simulink model "Foc_model_Matlab"  (R2024b)
settings: Solver=FixedStepDiscrete  StartTime=0.0  StopTime=2  RelTol=1e-3  EnableMultiTasking=on
PreLoadFcn:
  | mcb_pmsm_foc_hall_S32K144EVB_data;
InitFcn:
  | mbd_s32k_consistency_checks(bdroot(gcs));
model workspace (MAT data in the model file):
  IDC_OVERCURRENT = Simulink.Parameter
  IDC_OVERCURRENT.Value = 2.3
  IDC_OVERCURRENT.Complexity = 'real'
  IDC_OVERCURRENT.Dimensions = [1 1]
  IDC_OVERCURRENT.DataType = 'single'
  VDC_OVERVOLTAGE = Simulink.Parameter
  VDC_OVERVOLTAGE.Value = 16
  VDC_OVERVOLTAGE.Complexity = 'real'
  VDC_OVERVOLTAGE.Dimensions = [1 1]
  VDC_OVERVOLTAGE.DataType = 'single'
  VDC_UNDERVOLTAGE = Simulink.Parameter
  VDC_UNDERVOLTAGE.Value = 8
  VDC_UNDERVOLTAGE.Complexity = 'real'
  VDC_UNDERVOLTAGE.Dimensions = [1 1]
  VDC_UNDERVOLTAGE.DataType = 'single'
values from neighbouring files (symbols this model uses):
  Kcd = (1/pmsm.p)*(2*zeta1*wnd*pmsm.Ld)-pmsm.Rs    [Foc_data.m]
  Kcq = (2*zeta1*wnq*pmsm.Lq)-pmsm.Rs    [Foc_data.m]
  Kcs = (1/pmsm.p)*(2*zeta2*wns-(pmsm.B/pmsm.J))/((1.5*pmsm.p^2*pmsm.FluxPM)/pmsm.J)    [Foc_data.m]
  Kid = Kcd/t_id    [Foc_data.m]
  Kiq = Kcq/t_iq    [Foc_data.m]
  Kis = Kcs/t_is    [Foc_data.m]
  Ts = T_pwm * 2    (= 0.0001)    [Foc_data.m]
  Ts_motor = T_pwm    (= 5e-05)    [Foc_data.m]
  Ts_simulink = T_pwm    (= 5e-05)    [Foc_data.m]
  Ts_speed = 10*Ts    (= 0.001)    [Foc_data.m]
undefined symbols (not defined in the file or in its folder): External, inverter, LQFP, mcb_isCodeGenVar, mcb_isSimVar, One, PI_params, pmsm, PU_System, Shot, TRGMUX_PDB_TRIG
libraries: mbd_s32k1xx_ec_toolbox x39, mcbcontrolslib x9, simulink x6, mcbpositiondecoderlib x5, mbd_msd_ec_toolbox x5, hdlsllib x4, mcbplantlib x1, autolibpmsmexterior x1, SignalEditorBlockLib x1
(part 1 of 2)
Description:
  | Field-Oriented Control for PMSM with Hall sensor with MTRDEVSPNK144.
  | This Simulink model is designed to work with Linix 45ZWN24-40 Motor and validate
  | that the motor can be rotated in closed loop with Hall sensor in Mathworks model from Motor Control Blockset.
  | The main scope of the model is to validate that the motor can run using Field-Oriented Control with Hall sensor.
  | 
  | FEATURES:
  | - Use FreeMASTER pannel to control the speed,
  | - Measure the 3-phase sinusoidal currents with PWM-PDB-ADC synchronization,
  | - Measure the DC bus voltage and current with PWM-PDB-ADC synchronization,
  | - PI Speed, Flux and Torque Controllers, position observer using Hall sensor.
  | 
  | HW SETUP:
  | - Configure S32K144 board supply voltage: J107:2-3(over USB),
  | - Configure J9,J10 and J11 on MotorGD: 2-3 (mode PMSM),
  | - Rotate trimmer resistor R72 (placed Devkit-MotorGD) counter-clockwise at maximum,
  | - Connect the motor phases to MotorGD J13 connector
  |   (i.e. Linix 45ZWN24-40: phA-white/phB-blue/phC-green),
  | - Power on the kit via J7 connector with 12Vdc.
  | 
  | VALIDATION:
  | - Run "mcb_pmsm_hall_offset_S32K144EVB_NXP.mdl" model to find out the position offset and
  | update it in "mcb_pmsm_foc_hall_S32K144EVB_data.m" script, run this script,
  | - Build/Simulate the model,
  | - After reset or power on, the Green LED shall be ON,
  | - In case of a FAULT the Red LED will be ON,
  | - Open FreeMASTER project and connect to the target.
  | - The initial speed command is set to 450rpm and can be changed from FreeMaster project.
  | - Click on the ON/OFF button to start then the speed of the motor it can be
  | changed using Speed gauge.
  | 
  | NOTE:
  | - In case of fault (RED LED is ON), the remove fault cause and press RESET button
  | 
  | Copyright (c) 2021 NXP
  | version 1.0.0
settings Model: Creator=nxf40284  LastModifiedBy=diego
settings SolverCC: AlgebraicLoopSolver=TrustRegion
settings DataIOCC: ExternalInput=off  InitialState=off  LimitDataPoints=on  SaveFormat=Array  SaveOutput=off  SaveTime=off  ReturnWorkspaceOutputs=off
settings OptimizationCC: DefaultParameterBehavior=Inlined  UseFloatMulNetSlope=on  DefaultUnderspecifiedDataType=single  UseSpecifiedMinMax=on  EnhancedBackFolding=on  PassReuseOutputArgsAs=Individual arguments  ZeroExternalMemoryAtStartup=off  ZeroInternalMemoryAtStartup=off  NoFixptDivByZeroProtection=on  EfficientFloat2IntCast=on  EfficientTunableParamExpr=on
settings DebuggingCC: AlgebraicLoopMsg=error  ArtificialAlgebraicLoopMsg=error  SolverPrmCheckMsg=warning  InheritedTsInSrcMsg=none  MultiTaskDSMMsg=none  MultiTaskCondExecSysMsg=none  TasksWithSamePriorityMsg=none  SigSpecEnsureSampleTimeMsg=none  ParameterPrecisionLossMsg=none  ParameterTunabilityLossMsg=error  FcnCallInpInsideContextMsg=warning  UnconnectedInputMsg=error  UnconnectedOutputMsg=error  UnconnectedLineMsg=error  AllowSymbolicDim=off  StateNameClashWarn=warning  SFUnexpectedBacktrackingDiag=warning  SFNoUnconditionalDefaultTransitionDiag=warning  SFExecutionAtInitializationDiag=none  ArithmeticOperatorsInVariantConditions=warning
settings HardwareCC: ProdBitPerPointer=32  ProdBitPerSizeT=32  ProdBitPerPtrDiffT=32  ProdLargestAtomicInteger=Long  ProdLargestAtomicFloat=Double  ProdWordSize=32  ProdHWDeviceType=ARM Compatible->ARM Cortex
settings ModelReferenceCC: EnableRefExpFcnMdlSchedulingChecks=on
settings SFSimCC: MATLABDynamicMemAlloc=off
settings RTWCC: Description=Model Based Design Toolbox S32K1xx Code Generation Target  SystemTargetFile=mbd_s32k.tlc  MakeCommand=mbd_s32k_make_rtw COPY_MDLREF_INCLUDES=0  TemplateMakefile=mbd_s32k.tmf  GenerateReport=on  IncludeHyperlinkInReport=on  GenerateTraceInfo=on  GenerateTraceReport=on  GenerateTraceReportSl=on  GenerateTraceReportSf=on  GenerateTraceReportEml=on  GPUComputeCapability=3.5
settings CodeAppCC: ForceParamTrailComments=on  IgnoreCustomStorageClasses=off  OperatorAnnotations=on  SimulinkDataObjDesc=on  SFDataObjDesc=on  InsertBlockDesc=on  StateflowObjectComments=on
settings STFCustomTargetCC: MultiwordLength=256  CombineOutputUpdateFcns=on  ERTCustomFileBanners=on  SupportContinuousTime=off  SupportNonInlinedSFcns=off  RemoveResetFunc=on  MATLABClassNameForMDSCustomization=Simulink.SoftwareTarget.ERTCustomization  SystemTargetFile=mbd_s32k.tlc
settings ERTTargetCC: ParMdlRefBuildCompliant=off  CompOptLevelCompliant=off  ConcurrentExecutionCompliant=off  ModelStepFunctionPrototypeControlCompliant=off  CPPClassGenCompliant=off  UseToolchainInfoCompliant=off  ERTSrcFileBannerTemplate=mbd_ert_code_template.cgt  ERTHdrFileBannerTemplate=mbd_ert_code_template.cgt  ERTDataSrcFileTemplate=mbd_ert_code_template.cgt  ERTDataHdrFileTemplate=mbd_ert_code_template.cgt  ERTCustomFileTemplate=example_file_process.tlc  ConvertIfToSwitch=off  SuppressUnreachableDefaultCases=off  DynamicArrayContainerType=coder::array

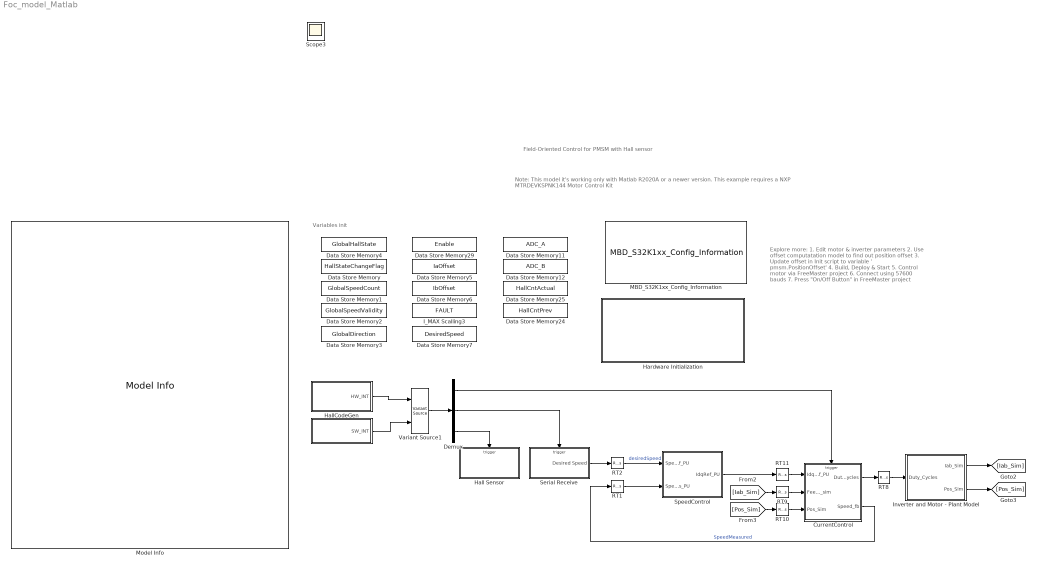
== system Foc_model_Matlab ==
  note: Variables init
  note: Field-Oriented Control for PMSM with Hall sensor
  note: Explore more:
      | 1. Edit motor & inverter parameters
      | 2. Use offset computatation model to
      | find out position offset
      | 3. Update offset in Init script to variable ' pmsm.PositionOffset'
      | 4. Build, Deploy & Start
      | 5. Control motor via FreeMaster project
      | 6. Connect using 57600 bauds
      | 7. Press "On/Off Button" in FreeMaster project
  note: Note: This model it's working only with Matlab R2020A or a newer version.
      | This example requires a NXP MTRDEVKSPNK144 Motor Control Kit
  " " : Subsystem
  CurrentControl : Subsystem
      settings: RTWSystemCode=Nonreusable function  RTWFcnNameOpts=Use subsystem name
  Data Store Memory : DataStoreMemory  DataStoreName=HallStateChangeFlag  ShowAdditionalParam=off  OutDataTypeStr=uint16
  Data Store Memory1 : DataStoreMemory  DataStoreName=GlobalSpeedCount  ShowAdditionalParam=off  OutDataTypeStr=uint16
  Data Store Memory11 : DataStoreMemory  DataStoreName=ADC_A  ShowAdditionalParam=off
  Data Store Memory12 : DataStoreMemory  DataStoreName=ADC_B  ShowAdditionalParam=off
  Data Store Memory2 : DataStoreMemory  DataStoreName=GlobalSpeedValidity  ShowAdditionalParam=off  OutDataTypeStr=uint16
  Data Store Memory24 : DataStoreMemory  DataStoreName=HallCntPrev  ReadBeforeWriteMsg=warning  WriteAfterWriteMsg=warning  WriteAfterReadMsg=warning  ShowAdditionalParam=off  OutDataTypeStr=uint16
  Data Store Memory25 : DataStoreMemory  DataStoreName=HallCntActual  ReadBeforeWriteMsg=warning  WriteAfterWriteMsg=warning  WriteAfterReadMsg=warning  ShowAdditionalParam=off  OutDataTypeStr=uint16
  Data Store Memory29 : DataStoreMemory  DataStoreName=Enable  ShowAdditionalParam=off  OutDataTypeStr=boolean
  Data Store Memory3 : DataStoreMemory  DataStoreName=GlobalDirection  ShowAdditionalParam=off  OutDataTypeStr=int16
  Data Store Memory4 : DataStoreMemory  DataStoreName=GlobalHallState  ShowAdditionalParam=off  OutDataTypeStr=uint32
  Data Store Memory5 : DataStoreMemory  DataStoreName=IaOffset  InitialValue=inverter.CtSensAOffset  ShowAdditionalParam=off  OutDataTypeStr=single
  Data Store Memory6 : DataStoreMemory  DataStoreName=IbOffset  InitialValue=inverter.CtSensBOffset  ShowAdditionalParam=off  OutDataTypeStr=single
  Data Store Memory7 : DataStoreMemory  DataStoreName=DesiredSpeed  ReadBeforeWriteMsg=warning  WriteAfterWriteMsg=warning  WriteAfterReadMsg=warning  InitialValue=450  ShowAdditionalParam=off  OutDataTypeStr=single
  Demux : Demux  Outputs=3
  Hall Sensor : Subsystem
  HallCodeGen : Subsystem
  Hardware Initialization : Subsystem  Priority=2
  I_MAX Scalling3 : DataStoreMemory  Priority=0  DataStoreName=FAULT  ReadBeforeWriteMsg=warning  WriteAfterWriteMsg=warning  WriteAfterReadMsg=warning  ShowAdditionalParam=off  OutDataTypeStr=boolean
  Inverter and Motor - Plant Model : Subsystem
  MBD_S32K1xx_Config_Information : mbd_s32k1xx_ec_toolbox/MBD_S32K1xx_Config_Information  Priority=1  mbdt_ver=0  disp_str=|  config_params=[]  mcu_target_name=S32K144  mcu_target_package=100-LQFP  mcu_target_sram_size=64KB  mcu_system_clock_freq=80  mcu_xtal_freq=External 8  mcu_steptick_timer=LPIT Channel 0  mcu_steptick_prio=15  ds_import_enable=on  target_compiler=GCC  target_memory=FLASH  gcc_target_compile_opts=-mcpu=cortex-m4 -mthumb -mfloat-abi=hard -mfpu=fpv4-sp-d16 -O1 -g -gstrict-dwarf  gcc_target_assemble_opts=-mcpu=cortex-m4 -mthumb -mfloat-abi=hard -mfpu=fpv4-sp-d16 -g  gcc_target_link_opts=-mcpu=cortex-m4 -mthumb -mfloat-abi=hard -mfpu=fpv4-sp-d16  gcc_target_default_lcf=on  gcc_target_user_lcf=S32K144_64_flash.ld  ghs_target_compile_opts=-cpu=cortexm4f -thumb -DARM_MATH_CM4 -fpu=vfpv4_d16 -fsingle -Ogeneral -Wundef -Wimplicit-int -Wshadow -Wtrigraphs --no_commons --gnu_asm -gnu99 -gdwarf-2 -G  ghs_target_assemble_opts=-cpu=cortexm4f -fpu=vfpv4_d16  ghs_target_link_opts=-cpu=cortexm4f -thumb -fpu=vfpv4_d16  ghs_target_default_lcf=on  ghs_target_user_lcf=S32K144_64_flash.ld  iar_target_compile_opts=--cpu=Cortex-M4F --thumb --fpu=VFPv4_sp -Ol -e --debug --dlib_config normal  iar_target_assemble_opts=--cpu Cortex-M4F --thumb --fpu VFPv4_sp  iar_target_link_opts=--no_exceptions --vfe --inline  iar_target_default_lcf=on  iar_target_user_lcf=S32K144_64_flash.icf  pil_download_enable=off  rbl_download_enable=on  rbl_start_delay=5000  rbl_download_interface=OpenSDA  rbl_restart_request=off  rbl_com_port=Custom  rbl_com_port_custom=COM1  pil_download_rate=57600  pil_opensda_drive=Custom  pil_opensda_drive_custom=D  pil_uart_instance=1  pil_uart_rx=PTC6: [LPUART1_RX | Receive]  pil_uart_tx=PTC7: [LPUART1_TX | Transmit]  FTM_PWM_PcrCheckEnDis=on  FTM_Input_Edge_Inputs_PcrCheckEnDis=on  FTM_Dual_Edge_Inputs_PcrCheckEnDis=on  FTM_Quadrature_Inputs_PcrCheckEnDis=on  FTM_Hall_Sensor_Inputs_PcrCheckEnDis=on  LPTMR_PcrCheckEnDis=on  PIT_PcrCheckEnDis=on  RTC_PcrCheckEnDis=on  FlexCAN_PcrCheckEnDis=on  LIN_PcrCheckEnDis=on  FlexIO_PcrCheckEnDis=on  LPI2C_PcrCheckEnDis=on  LPSPI_PcrCheckEnDis=on  LPUART_PcrCheckEnDis=on  CMP_PcrCheckEnDis=on  GPIO_OutputPcrCheckEnDis=on  GPIO_InputPcrCheckEnDis=on  SBC_PcrCheckEnDis=on  BMS_PcrCheckEnDis=on  AMMCLIB_PcrCheckEnDis=on  FM_PcrCheckEnDis=on  Profile_PcrCheckEnDis=on  ConfigParams_PcrCheckEnDis=on  ModelRef_PcrCheckEnDis=on  PDB0_PcrCheckEnDis=on  CSEc_PcrCheckEnDis=on  eDMA_PcrCheckEnDis=on  FLASH_PcrCheckEnDis=on  ADC_PcrCheckEnDis=on  WDOG_PcrCheckEnDis=on
      | Target : S32K144-64KB_SRAM
      | Package : 100-pin
      | System clock : 80 MHz
      | XTAL clock : External 8 MHz
      | Compiler : IAR
      | Target Type : FLASH
      | Download Code after build : off
      | Step Tick Interrupt Priority : 15
  Model Info : simulink/Model-Wide Utilities/Model Info  Frame=off  DisplayStringWithTags=|  HorizontalTextAlignment=Left  LeftAlignmentValue=0.02
      | Model Name: %<ModelName>
      | 
      | Description: %<Description>
  RT1 : RateTransition  Priority=2  Deterministic=off  OutPortSampleTime=Ts_speed
  RT10 : RateTransition  Deterministic=off  OutPortSampleTime=Ts
  RT11 : RateTransition  Deterministic=off  OutPortSampleTime=Ts
  RT2 : RateTransition  Priority=1  Deterministic=off  OutPortSampleTime=Ts_speed
  RT8 : RateTransition  Deterministic=off
  RT9 : RateTransition  Deterministic=off  OutPortSampleTime=Ts
  Serial Receive : Subsystem  SystemSampleTime=1e-3
  SpeedControl : Subsystem  TreatAsAtomicUnit=on  SystemSampleTime=Ts_speed
      settings: RTWSystemCode=Nonreusable function  RTWFcnNameOpts=Use subsystem name
  Variant Source1 : VariantSource
  Scope3 : Scope
  wires:
  " "/1(SW_INT) -> Variant Source1/2
  HallCodeGen/1(HW_INT) -> Variant Source1/1
  [Iab_Sim] -> RT9/1
  Serial Receive/1(Desired Speed) -> RT2/1
  RT9/1 -> CurrentControl/2(Feedbacks_sim)
  RT11/1 -> CurrentControl/1(Idq_ref_PU)
  [Pos_Sim] -> RT10/1
  RT10/1 -> CurrentControl/3(Pos_Sim)
  SpeedControl/1(IdqRef_PU) -> RT11/1
  RT2/1 -> SpeedControl/1(Speed_Ref_PU)  "desiredSpeed"
  CurrentControl/1(Duty Cycles) -> RT8/1
  RT8/1 -> Inverter and Motor - Plant Model/1(Duty_Cycles)
  Inverter and Motor - Plant Model/2(Pos_Sim) -> [Pos_Sim]
  Inverter and Motor - Plant Model/1(Iab_Sim) -> [Iab_Sim]
  RT1/1 -> SpeedControl/2(Speed_Meas_PU)
  CurrentControl/2(Speed_fb) -> RT1/1  "SpeedMeasured"
  Variant Source1/1 -> Demux/1
  Demux/3 -> Hall Sensor/Trigger
  Demux/2 -> Serial Receive/Trigger
  Demux/1 -> CurrentControl/Trigger

== system Foc_model_Matlab/  ==
  CurrentController_INT : simulink/Ports & Subsystems/Function-Call Generator  sample_time=Ts  numberOfIterations=1  DisallowWideOutput=off
  Hall_INT : simulink/Ports & Subsystems/Function-Call Generator  sample_time=Ts  numberOfIterations=1  DisallowWideOutput=off
  Mux : Mux  Inputs=3
  SCI_Rx_INT : simulink/Ports & Subsystems/Function-Call Generator  sample_time=0.1  numberOfIterations=1  DisallowWideOutput=off
  SW_INT : Outport
  wires:
  Mux/1 -> SW_INT/1
  CurrentController_INT/1 -> Mux/1
  Hall_INT/1 -> Mux/3
  SCI_Rx_INT/1 -> Mux/2

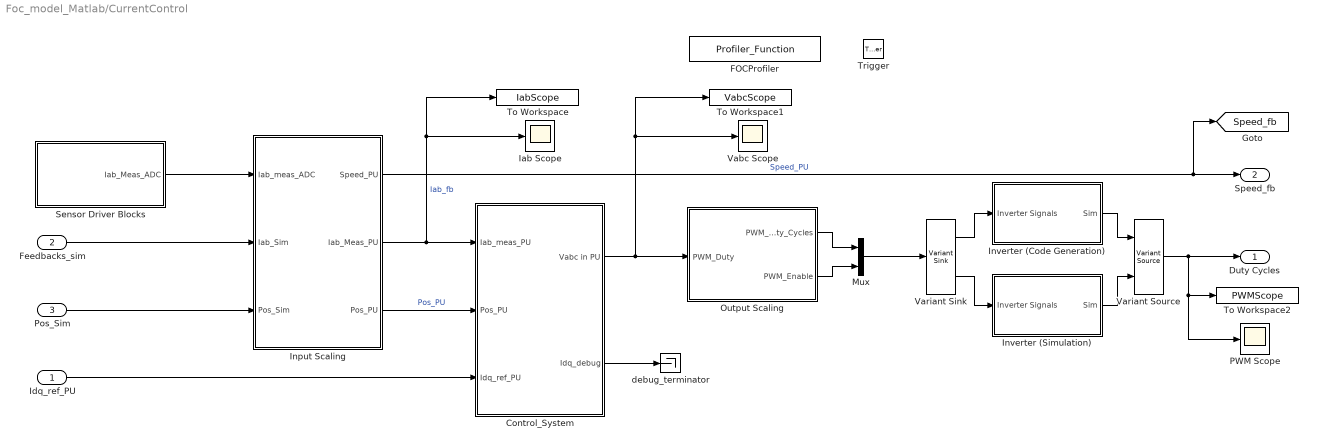
== system Foc_model_Matlab/CurrentControl ==
  Idq_ref_PU : Inport
  Feedbacks_sim : Inport  Port=2
  Pos_Sim : Inport  Port=3
  Trigger : TriggerPort  TriggerType=function-call  VariantControl=Variant
  Control_System : Subsystem  Priority=3
  FOCProfiler : mbd_s32k1xx_ec_toolbox/Utility Blocks/Profiler_Function  profile_indx=0
  Iab Scope : Scope
  Input Scaling : Subsystem  Priority=2  Variant=on  VariantControl=Variant1  PropagateVariantConditions=on
  Inverter (Code Generation) : Subsystem  Priority=5
  Inverter (Simulation) : Subsystem
  Mux : Mux  Inputs=2
  Output Scaling : Subsystem  Priority=4
  PWM Scope : Scope
  Sensor Driver Blocks : Subsystem  Variant=on
  To Workspace : ToWorkspace  VariableName=IabScope  SaveFormat=Structure With Time  SampleTime=-1
  To Workspace1 : ToWorkspace  VariableName=VabcScope  SaveFormat=Structure With Time  SampleTime=-1
  To Workspace2 : ToWorkspace  VariableName=PWMScope  SaveFormat=Structure With Time  SampleTime=-1
  Vabc Scope : Scope
  Variant Sink : VariantSink
  Variant Source : VariantSource
  debug_terminator : Terminator
  Duty Cycles : Outport  InitialOutput=0  VectorParamsAs1DForOutWhenUnconnected=off
  Speed_fb : Outport  Port=2  InitialOutput=0  VectorParamsAs1DForOutWhenUnconnected=off
  tag scope: Speed_fb=global
  wires:
  Sensor Driver Blocks/1(Iab_Meas_ADC) -> Input Scaling/1(Iab_meas_ADC)
  Control_System/1(Vabc in PU) -> To Workspace1/1, Vabc Scope/1, Output Scaling/1(PWM_Duty)
  Input Scaling/3(Pos_PU) -> Control_System/2(Pos_PU)  "Pos_PU"
  Idq_ref_PU/1 -> Control_System/3(Idq_ref_PU)
  Input Scaling/2(Iab_Meas_PU) -> To Workspace/1, Iab Scope/1, Control_System/1(Iab_meas_PU)  "Iab_fb"
  Pos_Sim/1 -> Input Scaling/3(Pos_Sim)
  Feedbacks_sim/1 -> Input Scaling/2(Iab_Sim)
  Output Scaling/1(PWM_Duty_Cycles) -> Mux/1
  Output Scaling/2(PWM_Enable) -> Mux/2
  Control_System/2(Idq_debug) -> debug_terminator/1
  Input Scaling/1(Speed_PU) -> [Speed_fb], Speed_fb/1  "Speed_PU"
  Variant Sink/1 -> Inverter (Code Generation)/1(Inverter Signals)
  Inverter (Code Generation)/1(Sim) -> Variant Source/1
  Inverter (Simulation)/1(Sim) -> Variant Source/2
  Variant Sink/2 -> Inverter (Simulation)/1(Inverter Signals)
  Mux/1 -> Variant Sink/1
  Variant Source/1 -> To Workspace2/1, PWM Scope/1, Duty Cycles/1

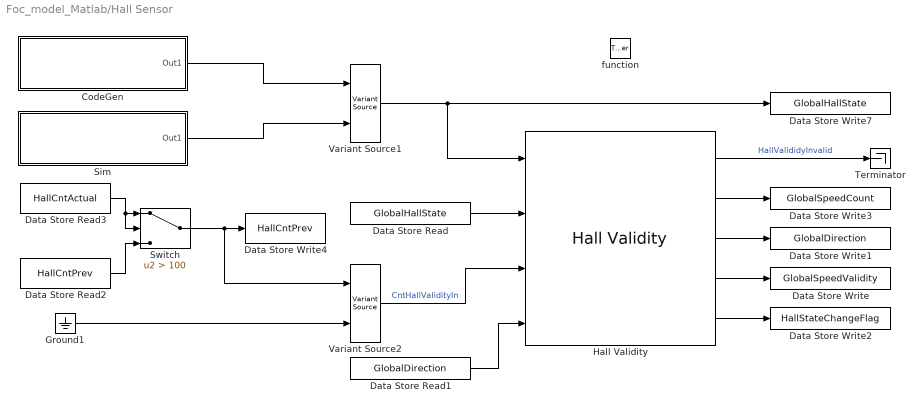
== system Foc_model_Matlab/Hall Sensor ==
  function : TriggerPort  TriggerType=function-call  VariantControl=Variant
  CodeGen : Subsystem
  Data Store Read : DataStoreRead  Priority=1  DataStoreName=GlobalHallState  IndexOptions=Index vector (dialog)  Indices=1  OutputSizes=1
  Data Store Read1 : DataStoreRead  DataStoreName=GlobalDirection  IndexOptions=Index vector (dialog)  Indices=1  OutputSizes=1
  Data Store Read2 : DataStoreRead  DataStoreName=HallCntPrev  IndexOptions=Index vector (dialog)  Indices=1  OutputSizes=1
  Data Store Read3 : DataStoreRead  DataStoreName=HallCntActual  IndexOptions=Index vector (dialog)  Indices=1  OutputSizes=1
  Data Store Write : DataStoreWrite  DataStoreName=GlobalSpeedValidity  IndexOptions=Index vector (dialog)  Indices=1  OutputSizes=1
  Data Store Write1 : DataStoreWrite  DataStoreName=GlobalDirection  IndexOptions=Index vector (dialog)  Indices=1  OutputSizes=1
  Data Store Write2 : DataStoreWrite  DataStoreName=HallStateChangeFlag  IndexOptions=Index vector (dialog)  Indices=1  OutputSizes=1
  Data Store Write3 : DataStoreWrite  DataStoreName=GlobalSpeedCount  IndexOptions=Index vector (dialog)  Indices=1  OutputSizes=1
  Data Store Write4 : DataStoreWrite  DataStoreName=HallCntPrev  IndexOptions=Index vector (dialog)  Indices=1  OutputSizes=1
  Data Store Write7 : DataStoreWrite  Priority=2  DataStoreName=GlobalHallState  IndexOptions=Index vector (dialog)  Indices=1  OutputSizes=1
  Ground1 : Ground
  Hall Validity : mcbpositiondecoderlib/Hall Validity  hallSequence=CBA  sequence=[6,4,5,1,3,2]  CounterSize=16 bits
  Sim : Subsystem
  Switch : Switch  Criteria=u2 > Threshold  Threshold=100  SaturateOnIntegerOverflow=off  InputSameDT=off
  Terminator : Terminator
  Variant Source1 : VariantSource
  Variant Source2 : VariantSource
  wires:
  Hall Validity/3 -> Data Store Write1/1
  Hall Validity/5 -> Data Store Write2/1
  Hall Validity/4 -> Data Store Write/1
  Data Store Read1/1 -> Hall Validity/4
  Hall Validity/2 -> Data Store Write3/1
  Data Store Read/1 -> Hall Validity/2
  Hall Validity/1 -> Terminator/1  "HallValididyInvalid"
  Variant Source1/1 -> Hall Validity/1, Data Store Write7/1
  Ground1/1 -> Variant Source2/2
  Switch/1 -> Variant Source2/1, Data Store Write4/1
  Sim/1(Out1) -> Variant Source1/2
  CodeGen/1(Out1) -> Variant Source1/1
  Data Store Read2/1 -> Switch/3
  Data Store Read3/1 -> Switch/2, Switch/1
  Variant Source2/1 -> Hall Validity/3  "CntHallValidityIn"

== system Foc_model_Matlab/HallCodeGen ==
  Data Store Write1 : DataStoreWrite  Priority=1  DataStoreName=HallCntActual  IndexOptions=Index vector (dialog)  Indices=1  OutputSizes=1
  FTM_Hall_Sensor : mbd_s32k1xx_ec_toolbox/Motor Control Blocks/FTM Blocks/FTM_Hall_Sensor  Priority=1  e_mode=Rising or Falling  prescaler=128  max_period=0.10486  isrlevel=5  mcuTargetUpdate=on  filter_en=off  filter_value=0  pinFtm1Ch1=PTA1: [FTM1_CH1 | FTM Channel]  pinFtm2Ch0=PTD10: [FTM2_CH0 | FTM Channel]  pinFtm2Ch1=PTD11: [FTM2_CH1 | FTM Channel]
  Mux : Mux  Inputs=3
  SCI_Rx_INT : simulink/Ports & Subsystems/Function-Call Generator  sample_time=0.1  numberOfIterations=1  DisallowWideOutput=off
  Subsystem2 : Subsystem  TreatAsAtomicUnit=on
  HW_INT : Outport
  wires:
  FTM_Hall_Sensor/2 -> Data Store Write1/1  "CntHall"
  Mux/1 -> HW_INT/1
  FTM_Hall_Sensor/1 -> Mux/3
  Subsystem2/1(FcnCall) -> Mux/1
  SCI_Rx_INT/1 -> Mux/2

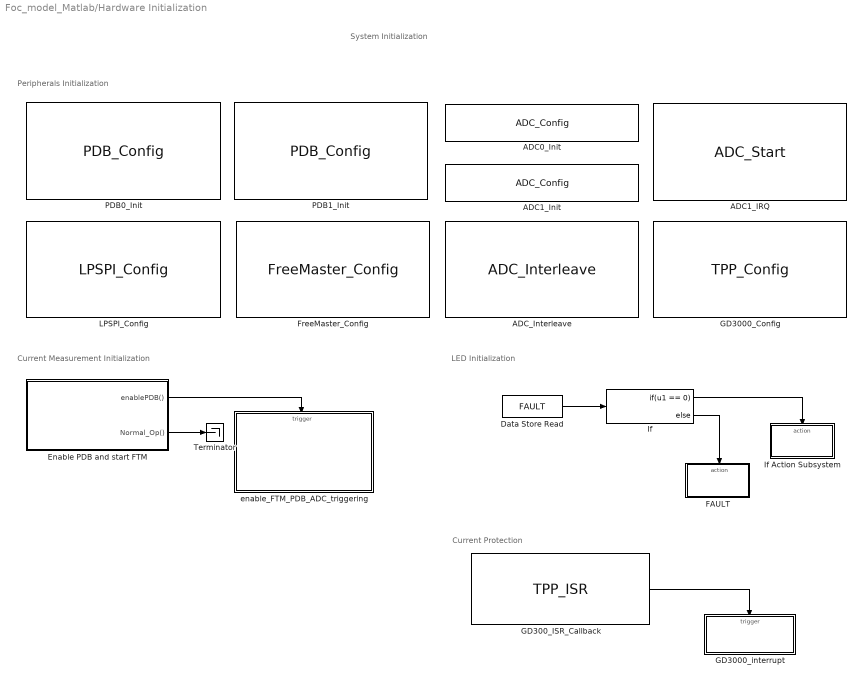
== system Foc_model_Matlab/Hardware Initialization ==
  note: Peripherals Initialization
  note: System Initialization
  note: Current Measurement Initialization
  note: LED Initialization
  note: Current Protection
  ADC0_Init : mbd_s32k1xx_ec_toolbox/Motor Control Blocks/ADC Blocks/ADC_Config  Priority=3  instance=0  mode=12-bit conversion  smplts=2  adiclk=alternate clock 1  adiv=input clock  show_adv_opts=on  pretrgsel=PDB pre-trigger  swpretrg=Disabled  adtrg=hardware  trgsel=PDB output  refsel=Vrefh and Vrefl  supply_monitoring=off  acfe=off  acfgt=off  acren=off  cv1=0  cv2=0  adco=off  avge=off  avgs=4 samples
  ADC1_IRQ : mbd_s32k1xx_ec_toolbox/Motor Control Blocks/ADC Blocks/ADC_Start  Priority=5  instance=1  adc_r=C  adc_chan=PTB16: [ADC1_SE15 | ADC Single Ended Input]  aien=on  mcuTargetUpdate=on
  ADC1_Init : mbd_s32k1xx_ec_toolbox/Motor Control Blocks/ADC Blocks/ADC_Config  Priority=4  instance=1  mode=12-bit conversion  smplts=2  adiclk=alternate clock 1  adiv=input clock  show_adv_opts=on  pretrgsel=PDB pre-trigger  swpretrg=Disabled  adtrg=hardware  trgsel=PDB output  refsel=Vrefh and Vrefl  supply_monitoring=off  acfe=off  acfgt=off  acren=off  cv1=0  cv2=0  adco=off  avge=off  avgs=4 samples
  ADC_Interleave : mbd_s32k1xx_ec_toolbox/Motor Control Blocks/ADC Blocks/ADC_Interleave  adcInterleavePins=PTB1 to ADC0_SE5 and ADC1_SE15  adcInterleaveInit=on
  Data Store Read : DataStoreRead  DataStoreName=FAULT  IndexOptions=Index vector (dialog)  Indices=1  OutputSizes=1
  Enable PDB and start FTM : Stateflow chart  TreatAsAtomicUnit=on
  FAULT : Subsystem  TreatAsAtomicUnit=on
  FreeMaster_Config : mbd_s32k1xx_ec_toolbox/Utility Blocks/FreeMaster_Config  interface=LPUART1  baudrate=57600  rxd=PTC6: [LPUART1_RX | Receive]  txd=PTC7: [LPUART1_TX | Transmit]  mode=Short Interrupt  isr_prio=14  show_adv_opts=on  use_scope=on  max_scope_vars=8  use_recorder=on  max_rec_vars=8  rec_buff_size=8192  rec_timebase=100 microseconds  comm_buffer_size_auto=on  comm_buffer_size=255  comm_rqueue_size_default=on  comm_rqueue_size=32
  GD3000_Config : mbd_msd_ec_toolbox/TPP/TPP_Config  Priority=1  tppInstance=0  desatMode=on  fullonMode=off  lockMode=off  overtempEvent=on  phaseEvent=off  desatEvent=off  framingEvent=on  vlsEvent=on  writeErrEvent=on  overcurrentEvent=on  resetEvent=on  mcuTppIntEn=off  prioInt=15  tppDeadtime=500  initTppNow=on  tppSpiInst=0  tppPwmModule=3  tppPair0_1=on  tppPair2_3=on  tppPair4_5=on  tppPair6_7=off  tppFirstChHS=on  tppEn1Pin=PTA2: [PTA2 | Port A I/O]  tppEn2Pin=PTA2: [PTA2 | Port A I/O]  tppRstPin=PTA3: [PTA3 | Port A I/O]  tppCsPin=PTB5: [PTB5 | Port B I/O]  tppIntPin=PTE10: [PTE10 | Port E I/O]
  GD3000_interrupt : Subsystem  TreatAsAtomicUnit=on
  "GD300_ISR_Callback " : mbd_msd_ec_toolbox/TPP/TPP_ISR  tppInstance=0
  If : If  IfExpression=u1 == 0
  If Action Subsystem : Subsystem  TreatAsAtomicUnit=on
  "LPSPI_Config " : mbd_s32k1xx_ec_toolbox/Communication Blocks/SPI Blocks/LPSPI_Config   InstanceNumber=0  Role=Master  BaudRate=1000000  ShowAdvanced=on  sin=PTB3: [LPSPI0_SIN | LPSPI Serial Data Input]  sout=PTB4: [LPSPI0_SOUT | LPSPI Serial Data Output]  sck=PTB2: [LPSPI0_SCK | LPSPI Serial Clock I/O]  pcs0=None  pcs1=PTB5: [LPSPI0_PCS1 | Peripheral Chip Select 1]  pcs2=None  pcs3=None  CPHA=1  CPOL=0  BitOrder=MSB first  TransferSize=8  WhichPCS=0  PCSPol=ActiveLow  ContinuousTransfer=off
  PDB0_Init : mbd_s32k1xx_ec_toolbox/Motor Control Blocks/PDB Blocks/PDB_Config  Priority=1  pdbModule=0  regScCont=One-Shot  regScTrgsel=External (TRGMUX_PDB_TRIG)  trgMuxSel=FTM3 Initialize Trigger  trgMuxSelPin=PTB5: [TRGMUX_IN0 | Trigger Mux Input]  regModModulus=5000  regScPrescaler=1  regScMult=1  regPoenPoen0=off  regPo0DlyDly1=0  regPo0DlyDly2=0  enable_pdb_init=off  show_adv_opts=on  regCh0C1En0=on  regCh0C1En1=off  regCh0C1En2=off  regCh0C1En3=off  regCh0C1En4=off  regCh0C1En5=off  regCh0C1En6=off  regCh0C1En7=off  regCh0C1Bb0=off  regCh0C1Bb1=off  regCh0C1Bb2=off  regCh0C1Bb3=off  regCh0C1Bb4=off  regCh0C1Bb5=off  regCh0C1Bb6=off  regCh0C1Bb7=off  regCh0C1Tos0=Pre-trigger is in delay mode  regCh0C1Tos1=Pre-trigger is in delay mode  regCh0C1Tos2=Pre-trigger is in delay mode  regCh0C1Tos3=Pre-trigger is in delay mode  regCh0C1Tos4=Pre-trigger is in delay mode  regCh0C1Tos5=Pre-trigger is in delay mode  regCh0C1Tos6=Pre-trigger is in delay mode  regCh0C1Tos7=Pre-trigger is in delay mode  regCh0DlyDly0=2000  regCh0DlyDly1=0  regCh0DlyDly2=0  regCh0DlyDly3=0  regCh0DlyDly4=0  regCh0DlyDly5=0  regCh0DlyDly6=0  regCh0DlyDly7=0  regCh1C1En0=off  regCh1C1En1=off  regCh1C1En2=off  regCh1C1En3=off  regCh1C1En4=off  regCh1C1En5=off  regCh1C1En6=off  regCh1C1En7=off  regCh1C1Bb0=off  regCh1C1Bb1=off  regCh1C1Bb2=off  regCh1C1Bb3=off  regCh1C1Bb4=off  regCh1C1Bb5=off  regCh1C1Bb6=off  regCh1C1Bb7=off  regCh1C1Tos0=Pre-trigger is in delay mode  regCh1C1Tos1=Pre-trigger is in delay mode  regCh1C1Tos2=Pre-trigger is in delay mode  regCh1C1Tos3=Pre-trigger is in delay mode  regCh1C1Tos4=Pre-trigger is in delay mode  regCh1C1Tos5=Pre-trigger is in delay mode  regCh1C1Tos6=Pre-trigger is in delay mode  regCh1C1Tos7=Pre-trigger is in delay mode  regCh1DlyDly0=0  regCh1DlyDly1=0  regCh1DlyDly2=0  regCh1DlyDly3=0  regCh1DlyDly4=0  regCh1DlyDly5=0  regCh1DlyDly6=0  regCh1DlyDly7=0
  PDB1_Init : mbd_s32k1xx_ec_toolbox/Motor Control Blocks/PDB Blocks/PDB_Config  Priority=2  pdbModule=1  regScCont=One-Shot  regScTrgsel=External (TRGMUX_PDB_TRIG)  trgMuxSel=FTM3 Initialize Trigger  trgMuxSelPin=PTB5: [TRGMUX_IN0 | Trigger Mux Input]  regModModulus=5000  regScPrescaler=1  regScMult=1  regPoenPoen0=off  regPo0DlyDly1=0  regPo0DlyDly2=0  enable_pdb_init=off  show_adv_opts=on  regCh0C1En0=on  regCh0C1En1=on  regCh0C1En2=on  regCh0C1En3=off  regCh0C1En4=off  regCh0C1En5=off  regCh0C1En6=off  regCh0C1En7=off  regCh0C1Bb0=off  regCh0C1Bb1=off  regCh0C1Bb2=off  regCh0C1Bb3=off  regCh0C1Bb4=off  regCh0C1Bb5=off  regCh0C1Bb6=off  regCh0C1Bb7=off  regCh0C1Tos0=Pre-trigger is in delay mode  regCh0C1Tos1=Pre-trigger is in delay mode  regCh0C1Tos2=Pre-trigger is in delay mode  regCh0C1Tos3=Pre-trigger is in delay mode  regCh0C1Tos4=Pre-trigger is in delay mode  regCh0C1Tos5=Pre-trigger is in delay mode  regCh0C1Tos6=Pre-trigger is in delay mode  regCh0C1Tos7=Pre-trigger is in delay mode  regCh0DlyDly0=0  regCh0DlyDly1=1000  regCh0DlyDly2=2000  regCh0DlyDly3=0  regCh0DlyDly4=0  regCh0DlyDly5=0  regCh0DlyDly6=0  regCh0DlyDly7=0  regCh1C1En0=off  regCh1C1En1=off  regCh1C1En2=off  regCh1C1En3=off  regCh1C1En4=off  regCh1C1En5=off  regCh1C1En6=off  regCh1C1En7=off  regCh1C1Bb0=off  regCh1C1Bb1=off  regCh1C1Bb2=off  regCh1C1Bb3=off  regCh1C1Bb4=off  regCh1C1Bb5=off  regCh1C1Bb6=off  regCh1C1Bb7=off  regCh1C1Tos0=Pre-trigger is in delay mode  regCh1C1Tos1=Pre-trigger is in delay mode  regCh1C1Tos2=Pre-trigger is in delay mode  regCh1C1Tos3=Pre-trigger is in delay mode  regCh1C1Tos4=Pre-trigger is in delay mode  regCh1C1Tos5=Pre-trigger is in delay mode  regCh1C1Tos6=Pre-trigger is in delay mode  regCh1C1Tos7=Pre-trigger is in delay mode  regCh1DlyDly0=0  regCh1DlyDly1=0  regCh1DlyDly2=0  regCh1DlyDly3=0  regCh1DlyDly4=0  regCh1DlyDly5=0  regCh1DlyDly6=0  regCh1DlyDly7=0
  Terminator : Terminator
  enable_FTM_PDB_ADC_triggering : Subsystem  TreatAsAtomicUnit=on
      settings: RTWSystemCode=Inline
  wires:
  Enable PDB and start FTM/1(enablePDB()) -> enable_FTM_PDB_ADC_triggering/Trigger
  Enable PDB and start FTM/2(Normal_Op()) -> Terminator/1
  Data Store Read/1 -> If/1
  If/1 -> If Action Subsystem/Action
  "GD300_ISR_Callback "/1 -> GD3000_interrupt/Trigger
  If/2 -> FAULT/Action

== system Foc_model_Matlab/Inverter and Motor - Plant Model ==
  Duty_Cycles : Inport
  Codegeneration : Subsystem
  Position Scope : Scope
  Simulation : Subsystem
  To Workspace : ToWorkspace  VariableName=PositionScope  SaveFormat=Structure With Time  SampleTime=-1
  Variant Sink : VariantSink
  Variant Source : VariantSource
  Variant Source1 : VariantSource
  Iab_Sim : Outport  VectorParamsAs1DForOutWhenUnconnected=off
  Pos_Sim : Outport  Port=2  VectorParamsAs1DForOutWhenUnconnected=off
  wires:
  Duty_Cycles/1 -> Variant Sink/1
  Variant Source/1 -> Iab_Sim/1
  Variant Source1/1 -> Pos_Sim/1
  Codegeneration/1(Iab_fb_Sim) -> Variant Source/1
  Codegeneration/2(Pos_fb_Sim) -> Variant Source1/1
  Variant Sink/1 -> Codegeneration/1(Duty_Cycles)
  Variant Sink/2 -> Simulation/1(Duty_Cycles)
  Simulation/1(Iab_fb_Sim) -> Variant Source/2
  Simulation/2(Pos_fb_Sim) -> Variant Source1/2, Position Scope/1, To Workspace/1

== system Foc_model_Matlab/Serial Receive ==
  function : TriggerPort  TriggerType=function-call  VariantControl=Variant
  Code Generation : Subsystem
  Data Store Write : DataStoreWrite  DataStoreName=Enable  IndexOptions=Index vector (dialog)  Indices=1  OutputSizes=1
  Data Type Conversion3 : DataTypeConversion  OutDataTypeStr=boolean  RndMeth=Simplest  SaturateOnIntegerOverflow=off
  Demux : Demux  Outputs=2
  Simulation : Subsystem
  Variant Source : VariantSource
  Desired Speed : Outport  VectorParamsAs1DForOutWhenUnconnected=off
  wires:
  Code Generation/1(Data) -> Variant Source/1
  Simulation/1(Data) -> Variant Source/2
  Variant Source/1 -> Demux/1
  Data Type Conversion3/1 -> Data Store Write/1
  Demux/2 -> Data Type Conversion3/1
  Demux/1 -> Desired Speed/1

== system Foc_model_Matlab/SpeedControl ==
  Speed_Ref_PU : Inport
  Speed_Meas_PU : Inport  Port=2
  FOCProfiler : mbd_s32k1xx_ec_toolbox/Utility Blocks/Profiler_Function  profile_indx=1
  Id_ref : Constant  Value=0  OutDataTypeStr=dataType  SampleTime=Ts_speed
  Mux : Mux  Inputs=2
  Mux1 : Mux  Inputs=2
  PI_Controller_Speed : Subsystem  Priority=2  TreatAsAtomicUnit=on
  Speed_Ref_Selector : Subsystem  Priority=1  TreatAsAtomicUnit=on
  To Workspace : ToWorkspace  VariableName=SpeedScope  SaveFormat=Structure With Time  SampleTime=-1
  IdqRef_PU : Outport  VectorParamsAs1DForOutWhenUnconnected=off
  wires:
  Speed_Meas_PU/1 -> Speed_Ref_Selector/2(Speed_Ref_Open), PI_Controller_Speed/2(N_fb), Mux/2  "Speed_fb"
  Id_ref/1 -> Mux1/1
  Mux1/1 -> IdqRef_PU/1
  Speed_Ref_PU/1 -> Speed_Ref_Selector/1(Speed_Ref_In)  "Speed_Ref_PU"
  Speed_Ref_Selector/1(Speed_Ref_PU) -> PI_Controller_Speed/1(N_ref), Mux/1  "Speed_Ref"
  PI_Controller_Speed/1(Iq_ref) -> Mux1/2  "Iq_ref"
  Mux/1 -> To Workspace/1

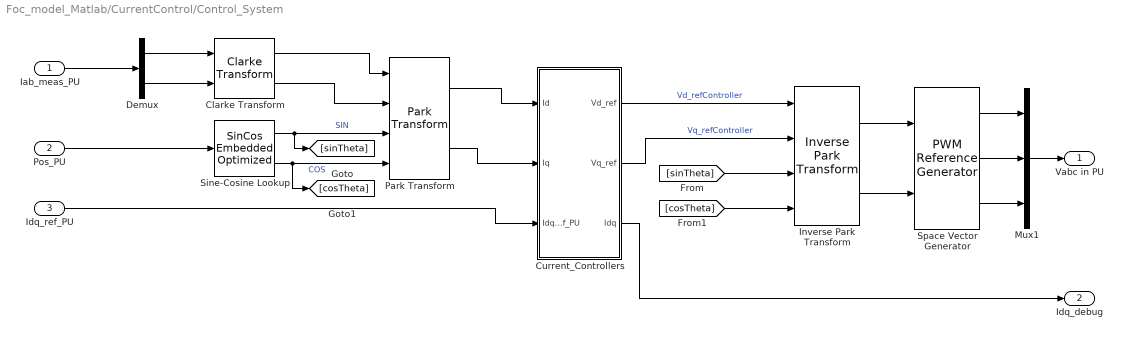
== system Foc_model_Matlab/CurrentControl/Control_System ==
  Iab_meas_PU : Inport
  Pos_PU : Inport  Port=2
  Idq_ref_PU : Inport  Port=3
  Clarke Transform : mcbcontrolslib/Clarke Transform  VariantControl=Variant2  PhaseInput=Two inputs  EnPowerInv=off
  Current_Controllers : Subsystem
  Demux : Demux  Outputs=2
  Inverse Park Transform : mcbcontrolslib/Inverse Park Transform  PhaseInput=Two inputs  AxisAlignment=D-axis  ThetaInput=Sine and Cosine electrical position  AngleInput=Per-unit  N_points=1024
  Mux1 : Mux  Inputs=3
  Park Transform : mcbcontrolslib/Park Transform  PhaseInput=Two inputs  AxisAlignment=D-axis  ThetaInput=Sine and Cosine electrical position  AngleInput=Per-unit  N_points=1024
  Sine-Cosine Lookup : mcbcontrolslib/SinCos Embedded Optimized  LabelModeActiveChoice=MCB_Sin  OptforProc=off  ApproximationMethod=None  UserApproxMethod=Lookup  ApproxStatus=None  InterpMethod=Linear point-slope  NumberOfDataPoints=16  NumberOfIterations=11  RemoveProtectionAgainstOutOfRangeInput=off  TableDataTypeStr=Inherit: Inherit via input  AngleInput=Per-unit  ThetaDataType=single  N_points=1024  DatatypeInput=Inherit from input  Datatype=Inherit: Same as input
  Space Vector Generator : mcbcontrolslib/PWM Reference Generator  inSignal=Valphabeta  modType=SVM: space vector modulation
  Vabc in PU : Outport  VectorParamsAs1DForOutWhenUnconnected=off
  Idq_debug : Outport  Port=2  VectorParamsAs1DForOutWhenUnconnected=off
  wires:
  Mux1/1 -> Vabc in PU/1
  [sinTheta] -> Inverse Park Transform/3
  Space Vector Generator/3 -> Mux1/3
  Space Vector Generator/1 -> Mux1/1
  Space Vector Generator/2 -> Mux1/2
  Idq_ref_PU/1 -> Current_Controllers/3(Idq_ref_PU)
  Iab_meas_PU/1 -> Demux/1
  Sine-Cosine Lookup/2 -> [cosTheta], Park Transform/4  "COS"
  Sine-Cosine Lookup/1 -> Park Transform/3, [sinTheta]  "SIN"
  Demux/1 -> Clarke Transform/1
  Demux/2 -> Clarke Transform/2
  Park Transform/2 -> Current_Controllers/2(Iq)
  Park Transform/1 -> Current_Controllers/1(Id)
  [cosTheta] -> Inverse Park Transform/4
  Current_Controllers/1(Vd_ref) -> Inverse Park Transform/1  "Vd_refController"
  Current_Controllers/2(Vq_ref) -> Inverse Park Transform/2  "Vq_refController"
  Pos_PU/1 -> Sine-Cosine Lookup/1
  Inverse Park Transform/1 -> Space Vector Generator/1
  Inverse Park Transform/2 -> Space Vector Generator/2
  Clarke Transform/1 -> Park Transform/1
  Clarke Transform/2 -> Park Transform/2
  Current_Controllers/3(Idq) -> Idq_debug/1

== system Foc_model_Matlab/CurrentControl/Input Scaling ==
  note: Variant control to pass plant simulated value for simulation and
      | ADC measured value for codegen.
  Iab_meas_ADC : Inport
  Iab_Sim : Inport  Port=2
  Pos_Sim : Inport  Port=3
  Read_Sensor (codegen) : Subsystem  VariantControl=mcb_isCodeGenVar()
  Read_Sensor (sim) : Subsystem  VariantControl=mcb_isSimVar()
  Speed_PU : Outport  VectorParamsAs1DForOutWhenUnconnected=off
  Iab_Meas_PU : Outport  Port=2  VectorParamsAs1DForOutWhenUnconnected=off
  Pos_PU : Outport  Port=3  VectorParamsAs1DForOutWhenUnconnected=off

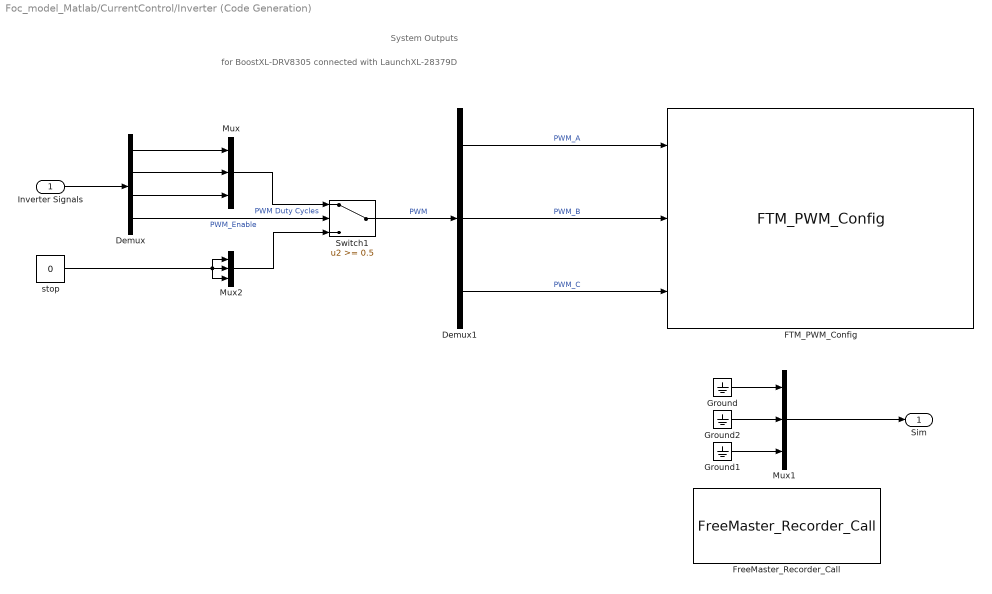
== system Foc_model_Matlab/CurrentControl/Inverter (Code Generation) ==
  note: for BoostXL-DRV8305 connected with LaunchXL-28379D
  note: System Outputs
  Inverter Signals : Inport
  Demux : Demux
  Demux1 : Demux  Outputs=3
  FTM_PWM_Config : mbd_s32k1xx_ec_toolbox/Motor Control Blocks/FTM Blocks/FTM_PWM_Config  ftmModule=3  ftmMode=Center-Aligned PWM  ftmSourceClock=80 MHz  swcontrol_enable=off  chan0En=on  chan0Type=Complementary  chan2En=on  chan2Type=Complementary  chan4En=on  chan4Type=Complementary  chan6En=off  chan6Type=Independent  ftmPwmUnits=Hz  outFrequency=20000  ftmPeriod=4000  ftmPrescaler=Divide by 1  deadtimeUnits=Nanoseconds  deadtimeNs=0  deadtimeTicks=0  deadtimePrescaler=Divide by 1  dutyCycleCh0=0  dutyCycleCh1=0  dutyCycleCh2=0  dutyCycleCh3=0  dutyCycleCh4=0  dutyCycleCh5=0  dutyCycleCh6=0.25  dutyCycleCh7=0.25  dutyCycleSim=off  startAfterInit=off  showAdvOpt=on  pinFtmCh0=PTB8: [FTM3_CH0 | FTM Channel]  pinFtmCh1=PTB9: [FTM3_CH1 | FTM Channel]  pinPolCh0=Active Low  pinPolCh1=Active Low  outputComplem0=Main duplicated  outputLevel0=High  outputLevel1=Low  pinFtmCh2=PTB10: [FTM3_CH2 | FTM Channel]  pinFtmCh3=PTB11: [FTM3_CH3 | FTM Channel]  pinPolCh2=Active Low  pinPolCh3=Active Low  outputComplem2=Main duplicated  outputLevel2=High  outputLevel3=Low  pinFtmCh4=PTC10: [FTM3_CH4 | FTM Channel]  pinFtmCh5=PTC11: [FTM3_CH5 | FTM Channel]  pinPolCh4=Active Low  pinPolCh5=Active Low  outputComplem4=Main duplicated  outputLevel4=High  outputLevel5=Low  pinFtmCh6=PTC12: [FTM3_CH6 | FTM Channel]  pinFtmCh7=None  pinPolCh6=Active Low  pinPolCh7=Active Low  outputComplem6=Main duplicated  outputLevel6=Low  outputLevel7=Low  initTrigger=off  chTrigger0=off  chTrigger1=off  chTrigger2=off  chTrigger3=off  chTrigger4=off  chTrigger5=off  chTrigger6=off  chTrigger7=off  mcuTargetUpdate=on  pwmSyncTrg=Software trigger  pwmSyncHwRouting=TRGMUX_FTM7  pwmSyncTrg0=off  pwmSyncTrg1=off  pwmSyncTrg2=off  pwmSyncAutoClear=off  pwmSyncMinLoad=off  pwmSyncMaxLoad=on  pwmSyncInvert=PWM Syncronization  pwmSyncOutControl=PWM Syncronization  pwmSyncOutMask=PWM Syncronization  pwmSyncCounterInitial=PWM Syncronization  pwmSyncPoints=Wait Loading Points  reloadEnable=off  reloadPriority=15  reloadHalfCycle=off  reloadHCR=0  reloadFrequency=0  chnMatch0=off  chnMatch1=off  chnMatch2=off  chnMatch3=off  chnMatch4=off  chnMatch5=off  chnMatch6=off  chnMatch7=off  pwmFaultProtection=off  pwmFaultInterrupt=off  pwmFaultClearing=Fault control disabled  pwmFaultPinState=Safe Value  pwmFaultFilterValue=0  pwmFaultPriority=15  fault_disen_0=off  fault_filter_0=off  fault_polarity_0=Active High  fault_disen_1=off  fault_filter_1=off  fault_polarity_1=Active high  fault_disen_2=off  fault_filter_2=off  fault_polarity_2=Active high  fault_disen_3=off  fault_filter_3=off  fault_polarity_3=Active high  fault_pin_0=None  fault_pin_1=None  fault_pin_2=None  fault_pin_3=None
  FreeMaster_Recorder_Call : mbd_s32k1xx_ec_toolbox/Utility Blocks/FreeMaster_Recorder_Call
  Ground : Ground
  Ground1 : Ground
  Ground2 : Ground
  Mux : Mux  Inputs=3
  Mux1 : Mux  Inputs=3
  Mux2 : Mux  Inputs=3
  Switch1 : Switch  Threshold=0.5  SaturateOnIntegerOverflow=off  InputSameDT=off
  stop : Constant  Value=0  OutDataTypeStr=Inherit: Inherit via back propagation
  Sim : Outport  VectorParamsAs1DForOutWhenUnconnected=off
  wires:
  Mux/1 -> Switch1/1  "PWM Duty Cycles"
  Demux/1 -> Mux/1
  Demux/3 -> Mux/3
  stop/1 -> Mux2/3, Mux2/2, Mux2/1
  Mux2/1 -> Switch1/3
  Inverter Signals/1 -> Demux/1
  Demux/2 -> Mux/2
  Demux/4 -> Switch1/2  "PWM_Enable"
  Switch1/1 -> Demux1/1  "PWM"
  Demux1/1 -> FTM_PWM_Config/1  "PWM_A"
  Demux1/2 -> FTM_PWM_Config/2  "PWM_B"
  Demux1/3 -> FTM_PWM_Config/3  "PWM_C"
  Ground2/1 -> Mux1/2
  Ground1/1 -> Mux1/3
  Ground/1 -> Mux1/1
  Mux1/1 -> Sim/1

== system Foc_model_Matlab/CurrentControl/Inverter (Simulation) ==
  Inverter Signals : Inport
  Data Type Duplicate : DataTypeDuplicate
  Demux : Demux
  Mux : Mux  Inputs=3
  Mux2 : Mux  Inputs=3
  Switch1 : Switch  Threshold=0.5  RndMeth=Simplest  SaturateOnIntegerOverflow=off  InputSameDT=off
  stop : Constant  Value=0  OutDataTypeStr=Inherit: Inherit via back propagation
  Sim : Outport  VectorParamsAs1DForOutWhenUnconnected=off
  wires:
  stop/1 -> Data Type Duplicate/2, Mux2/1, Mux2/3, Mux2/2
  Mux2/1 -> Switch1/3
  Switch1/1 -> Sim/1
  Inverter Signals/1 -> Demux/1
  Demux/4 -> Switch1/2  "PWM Enable"
  Mux/1 -> Data Type Duplicate/1, Switch1/1  "PWM Duty Cycles"
  Demux/1 -> Mux/1
  Demux/2 -> Mux/2
  Demux/3 -> Mux/3

== system Foc_model_Matlab/CurrentControl/Output Scaling ==
  PWM_Duty : Inport
  Constant1 : Constant  OutDataTypeStr=Inherit: Inherit via back propagation
  Data Type Conversion : DataTypeConversion  OutDataTypeStr=dataType  SaturateOnIntegerOverflow=off  RndMeth=Floor
  Enable : DataStoreRead  DataStoreName=Enable  IndexOptions=Index vector (dialog)  Indices=1  OutputSizes=1
  Gain : Gain  Gain=0.5  OutDataTypeStr=Inherit: Inherit via back propagation  RndMeth=Simplest
  Sum1 : Sum  Inputs=|++  RndMeth=Simplest
  PWM_Duty_Cycles : Outport
  PWM_Enable : Outport  Port=2
  wires:
  Enable/1 -> Data Type Conversion/1  "PWM_En"
  Data Type Conversion/1 -> PWM_Enable/1
  Gain/1 -> PWM_Duty_Cycles/1  "PWM_Duty_Cycles"
  Sum1/1 -> Gain/1
  Constant1/1 -> Sum1/2
  PWM_Duty/1 -> Sum1/1

== system Foc_model_Matlab/CurrentControl/Sensor Driver Blocks ==
  Sensor Driver Blocks (codegen) : Subsystem  VariantControl=mcb_isCodeGenVar()
  Sensor Driver Blocks (sim) : Subsystem  VariantControl=mcb_isSimVar()
  Iab_Meas_ADC : Outport

== system Foc_model_Matlab/Hall Sensor/CodeGen ==
  Add1 : Sum  Inputs=+++  OutDataTypeStr=Inherit: Inherit via back propagation
  Bit Shift : hdlsllib/Logic and Bit Operations/Bit Shift  mode=Shift Left Logical  N=2
  Bit Shift1 : hdlsllib/Logic and Bit Operations/Bit Shift  mode=Shift Left Logical  N=1
  Data Type Conversion2 : DataTypeConversion  OutDataTypeStr=uint32  SaturateOnIntegerOverflow=off  RndMeth=Floor
  Data Type Conversion3 : DataTypeConversion  OutDataTypeStr=uint32  SaturateOnIntegerOverflow=off  RndMeth=Floor
  Data Type Conversion6 : DataTypeConversion  OutDataTypeStr=uint32  SaturateOnIntegerOverflow=off  RndMeth=Floor
  Digital_Input_HALL_A : mbd_s32k1xx_ec_toolbox/GPIO Blocks/Digital_Input  gpio_pin=PTA1: [PTA1 | Port A I/O]  pull_resistor=None  passive_filter=off
  Digital_Input_HALL_B : mbd_s32k1xx_ec_toolbox/GPIO Blocks/Digital_Input  gpio_pin=PTD10: [PTD10 | Port D I/O]  pull_resistor=None  passive_filter=off
  Digital_Input_HALL_C : mbd_s32k1xx_ec_toolbox/GPIO Blocks/Digital_Input  gpio_pin=PTD11: [PTD11 | Port D I/O]  pull_resistor=None  passive_filter=off
  Out1 : Outport
  wires:
  Bit Shift1/1 -> Add1/2  "HALL_B"
  Digital_Input_HALL_B/1 -> Data Type Conversion2/1
  Add1/1 -> Out1/1
  Data Type Conversion6/1 -> Add1/3  "HALL_C"
  Digital_Input_HALL_A/1 -> Data Type Conversion3/1
  Data Type Conversion2/1 -> Bit Shift1/1
  Bit Shift/1 -> Add1/1  "HALL_A"
  Digital_Input_HALL_C/1 -> Data Type Conversion6/1
  Data Type Conversion3/1 -> Bit Shift/1

== system Foc_model_Matlab/Hall Sensor/Sim ==
  Data Type Conversion1 : DataTypeConversion  OutDataTypeStr=uint32  SaturateOnIntegerOverflow=off  RndMeth=Floor
  Ground : Ground
  Out1 : Outport
  wires:
  Ground/1 -> Data Type Conversion1/1
  Data Type Conversion1/1 -> Out1/1

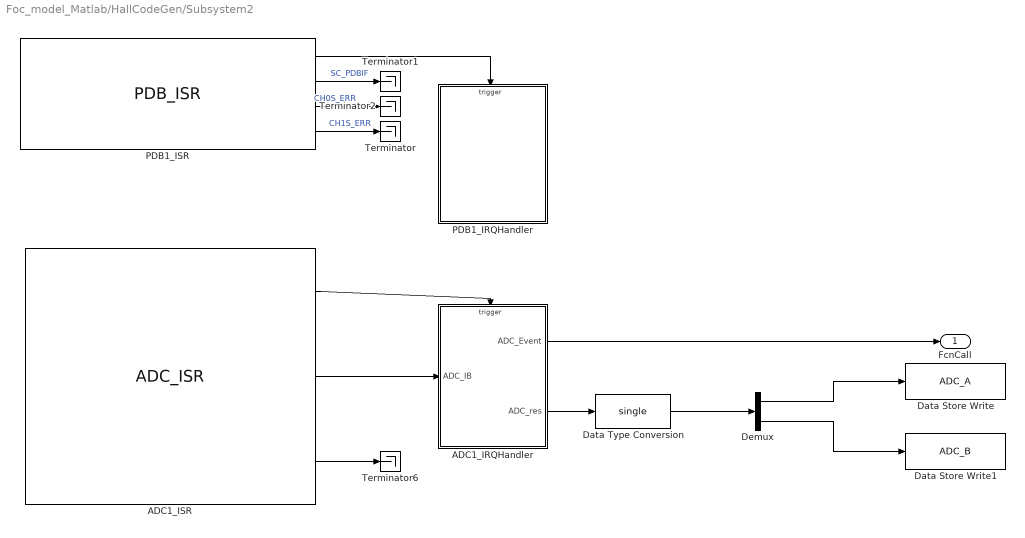
== system Foc_model_Matlab/HallCodeGen/Subsystem2 ==
  ADC1_IRQHandler : Subsystem  TreatAsAtomicUnit=on
  ADC1_ISR : mbd_s32k1xx_ec_toolbox/Motor Control Blocks/ADC Blocks/ADC_ISR  instance=1  pri=5  sc1n=C
  Data Store Write : DataStoreWrite  DataStoreName=ADC_A  IndexOptions=Index vector (dialog)  Indices=1  OutputSizes=1
  Data Store Write1 : DataStoreWrite  DataStoreName=ADC_B  IndexOptions=Index vector (dialog)  Indices=1  OutputSizes=1
  Data Type Conversion : DataTypeConversion  OutDataTypeStr=single  SaturateOnIntegerOverflow=off  RndMeth=Floor
  Demux : Demux  Outputs=2
  PDB1_IRQHandler : Subsystem  TreatAsAtomicUnit=on
  PDB1_ISR : mbd_s32k1xx_ec_toolbox/Motor Control Blocks/PDB Blocks/PDB_ISR  Priority=8  pdbModule=0  prioInterrupt=6  regScPdbie=on  regScPdbeie=off  regIdlyIdly=4999
  Terminator{,1..2,6} (4 alike) : Terminator
  FcnCall : Outport  VectorParamsAs1DForOutWhenUnconnected=off
  wires:
  ADC1_IRQHandler/2(ADC_res) -> Data Type Conversion/1
  PDB1_ISR/1 -> PDB1_IRQHandler/Trigger
  PDB1_ISR/3 -> Terminator2/1  "CH0S_ERR"
  PDB1_ISR/4 -> Terminator/1  "CH1S_ERR"
  ADC1_ISR/1 -> ADC1_IRQHandler/Trigger
  PDB1_ISR/2 -> Terminator1/1  "SC_PDBIF"
  ADC1_ISR/2 -> ADC1_IRQHandler/1(ADC_IB)
  ADC1_IRQHandler/1(ADC_Event) -> FcnCall/1
  ADC1_ISR/3 -> Terminator6/1
  Demux/2 -> Data Store Write1/1
  Data Type Conversion/1 -> Demux/1
  Demux/1 -> Data Store Write/1

== system Foc_model_Matlab/Hardware Initialization/FAULT ==
  Action Port : ActionPort  ActionPortLabel=else
  LED_GREEN : mbd_s32k1xx_ec_toolbox/GPIO Blocks/Digital_Output  gpio_pin=PTD16: [PTD16 | Port D I/O]  init_val=Low  drive_strength=Low
  LED_RED : mbd_s32k1xx_ec_toolbox/GPIO Blocks/Digital_Output  gpio_pin=PTD15: [PTD15 | Port D I/O]  init_val=Low  drive_strength=Low
  OFF : Constant  OutDataTypeStr=boolean
  ON : Constant  Value=0  OutDataTypeStr=boolean
  wires:
  OFF/1 -> LED_GREEN/1
  ON/1 -> LED_RED/1

== system Foc_model_Matlab/Hardware Initialization/GD3000_interrupt ==
  function : TriggerPort  TriggerType=function-call  VariantControl=Variant
  FAULT_write : DataStoreWrite  DataStoreName=FAULT  IndexOptions=Index vector (dialog)  Indices=1  OutputSizes=1
  FTM_PWM_Disable_Enable : mbd_s32k1xx_ec_toolbox/Motor Control Blocks/FTM Blocks/FTM_PWM_Disable_Enable  ftmModule=3  action=Disable
  NOK : Constant  OutDataTypeStr=boolean
  TPP_Functional_Mode : mbd_msd_ec_toolbox/TPP/TPP_Functional_Mode  tppInstance=0  action=Sleep
  wires:
  NOK/1 -> FAULT_write/1

== system Foc_model_Matlab/Hardware Initialization/If Action Subsystem ==
  Action Port : ActionPort  ActionPortLabel=if(u1 == 0)
  LED_GREEN : Constant  Value=0  OutDataTypeStr=boolean  SampleTime=-1
  LED_GREEN_ON : mbd_s32k1xx_ec_toolbox/GPIO Blocks/Digital_Output  gpio_pin=PTD16: [PTD16 | Port D I/O]  init_val=Low  drive_strength=Low
  LED_RED : Constant  OutDataTypeStr=boolean  SampleTime=-1
  LED_RED_OFF : mbd_s32k1xx_ec_toolbox/GPIO Blocks/Digital_Output  gpio_pin=PTD15: [PTD15 | Port D I/O]  init_val=Low  drive_strength=Low
  wires:
  LED_GREEN/1 -> LED_GREEN_ON/1
  LED_RED/1 -> LED_RED_OFF/1

== system Foc_model_Matlab/Hardware Initialization/enable_FTM_PDB_ADC_triggering ==
  function : TriggerPort  TriggerType=function-call  VariantControl=(inherit)
  Custom code to reload the PDB value : Subsystem  Priority=6  mask(System Outputs){ShowInLibBrowser=0}
      mask prompts: ShowInLibBrowser "Simulink:masks:CustCodeMaskParam1_MP"
      settings: CopyFcn=cccopyfcn(gcb)  OpenFcn=ccopenfcn('System Outputs Function')
      mask Help: eval('feval(''rtwprivate'',''rtwhelpview'',''rtw_sys_outputs_block'')');
      mask Display: disp('System\nOutputs');
  FTM_Init_Trigger_Disable_Enable : mbd_s32k1xx_ec_toolbox/Motor Control Blocks/FTM Blocks/FTM_Init_Trigger_Disable_Enable  Priority=3  ftmModule=3  action=Enable
  FTM_PWM_Disable_Enable : mbd_s32k1xx_ec_toolbox/Motor Control Blocks/FTM Blocks/FTM_PWM_Disable_Enable  Priority=1  ftmModule=3  action=Enable
  PDB0_Enable : mbd_s32k1xx_ec_toolbox/Motor Control Blocks/PDB Blocks/PDB_Enable  Priority=4  pdbModule=0  pdbAction=Enable
  PDB1_Enable : mbd_s32k1xx_ec_toolbox/Motor Control Blocks/PDB Blocks/PDB_Enable  Priority=5  pdbModule=1  pdbAction=Enable
  TPP_ISR_Enable_Disable : mbd_msd_ec_toolbox/TPP/TPP_ISR_Enable_Disable  Priority=7  tppInstance=0  mcuTppIntEn=on  prioInt=15

== system Foc_model_Matlab/Inverter and Motor - Plant Model/Codegeneration ==
  Duty_Cycles : Inport
  Ground : Ground
  Ground1 : Ground
  Terminator : Terminator
  Iab_fb_Sim : Outport  VectorParamsAs1DForOutWhenUnconnected=off
  Pos_fb_Sim : Outport  Port=2  VectorParamsAs1DForOutWhenUnconnected=off
  wires:
  Duty_Cycles/1 -> Terminator/1
  Ground/1 -> Iab_fb_Sim/1
  Ground1/1 -> Pos_fb_Sim/1

== system Foc_model_Matlab/Inverter and Motor - Plant Model/Simulation ==
  Duty_Cycles : Inport
  Average Inverter : Subsystem
  Load_Profile (Torque) : Subsystem
  RT1 : RateTransition  Deterministic=off  OutPortSampleTime=Ts_simulink
  RT3 : RateTransition  Deterministic=off  OutPortSampleTime=Ts_simulink
  Rate Transition : RateTransition  Deterministic=off  OutPortSampleTime=Ts_motor
  Rate Transition1 : RateTransition  Deterministic=off  OutPortSampleTime=Ts_motor
  Sensor_Measurements : Subsystem
  Surface Mount PMSM : autolibpmsmexterior/Surface Mount PMSM  port_config=Torque  sim_type=Discrete  Ts=Ts_motor  FilePath=surfacepmsm_motordata.m  P=pmsm.p  Rs=pmsm.Rs + inverter.R_board  Ldq_=pmsm.Ld  KConstText=Permanent flux linkage constant (lambda_pm):  lambda_pm=pmsm.FluxPM  Ke=159.9771  Kt=1.323  mechanical=[pmsm.J, pmsm.B, 0]  idq0=[0 0]  theta_init=0  omega_init=0  KConst=pmsm.FluxPM  lambda_pm_calc=pmsm.FluxPM  RefBlkName='autolibpmsmexterior/Surface Mount PMSM'  aMode=5  Ldq="[0.0006      0.0006]"
  Terminator : Terminator
  Iab_fb_Sim : Outport  VectorParamsAs1DForOutWhenUnconnected=off
  Pos_fb_Sim : Outport  Port=2  VectorParamsAs1DForOutWhenUnconnected=off
  wires:
  RT1/1 -> Sensor_Measurements/2(PhaseCurr)
  Surface Mount PMSM/3 -> Terminator/1
  Average Inverter/1(Vabc) -> Rate Transition/1
  Load_Profile (Torque)/1(Load_Trq) -> Rate Transition1/1
  Surface Mount PMSM/2 -> RT1/1  "Iabc"
  RT3/1 -> Sensor_Measurements/1(Info)
  Surface Mount PMSM/1 -> RT3/1
  Rate Transition1/1 -> Surface Mount PMSM/1
  Rate Transition/1 -> Surface Mount PMSM/2
  Duty_Cycles/1 -> Average Inverter/1(Duty_abc)
  Sensor_Measurements/1(Iab_fb) -> Iab_fb_Sim/1
  Sensor_Measurements/2(Pos_fb) -> Pos_fb_Sim/1

== system Foc_model_Matlab/Serial Receive/Code Generation ==
  Data Store Read2 : DataStoreRead  DataStoreName=DesiredSpeed  IndexOptions=Index vector (dialog)  Indices=1  OutputSizes=1
  Data Store Read3 : DataStoreRead  DataStoreName=Enable  IndexOptions=Index vector (dialog)  Indices=1  OutputSizes=1
  Data Type Conversion5 : DataTypeConversion  OutDataTypeStr=single  RndMeth=Simplest  SaturateOnIntegerOverflow=off
  Mux1 : Mux  Inputs=2
  rpm2PU : Gain  Gain=1/pmsm.N_max  RndMeth=Simplest
  Data : Outport
  wires:
  Data Store Read3/1 -> Data Type Conversion5/1
  Data Type Conversion5/1 -> Mux1/2
  rpm2PU/1 -> Mux1/1
  Mux1/1 -> Data/1
  Data Store Read2/1 -> rpm2PU/1

== system Foc_model_Matlab/Serial Receive/Simulation ==
  Cast To Single : DataTypeConversion  Commented=on  OutDataTypeStr=single  SaturateOnIntegerOverflow=off  RndMeth=Floor
  Gain : Gain  Gain=1/pmsm.N_max
  Mux2 : Mux  Inputs=2
  Signal Editor : SignalEditorBlockLib/Signal Editor  Commented=on  FileName=SpeedController.mat  ActiveScenario=SpeedController  ActiveSignal=Step  IsBus=off  OutputBusObjectStr=Bus: BusObject  SampleTime=-1  Interpolate=off  OutputAfterFinalValue=Holding final value  Unit=inherit  PreserveSignalName=on  ApplySigPropsToAllScenarios=on  ApplySigPropsToAllSignals=off
  Speed_Ref_Final (rpm)1 : Constant  Value=0.8*pmsm.N_max  OutDataTypeStr=dataType  SampleTime=-1
  Speed_Ref_Init (rpm)1 : Step  Time=0  OutDataTypeStr=single
  rotor2elec : Gain  Commented=through  Gain=pmsm.p
  rpm2rad/s : Gain  Commented=through  Gain=2*pi/60
  Data : Outport
  wires:
  Mux2/1 -> Data/1
  Speed_Ref_Init (rpm)1/1 -> Mux2/2
  Signal Editor/1 -> Cast To Single/1
  Gain/1 -> Mux2/1
  Speed_Ref_Final (rpm)1/1 -> Gain/1
